simulink model "Model_CzasKroku"  (R2020b)
settings: Solver=VariableStepAuto  StartTime=0.0  StopTime=60  RelTol=1e-3
values from neighbouring files (symbols this model uses):
  g = 9.80665    [Strojenie_LQR_CzasKroku.m]    (also in Strojenie_LQR_Sila.m)
  K = lqr(A,B,Q,R)    [Strojenie_LQR_CzasKroku.m]    (also in Strojenie_LQR_Sila.m)
  L = 0.25    [Strojenie_LQR_CzasKroku.m]    (also in Strojenie_LQR_Sila.m)
  M = 1.5    [Strojenie_LQR_CzasKroku.m]    (also in Strojenie_LQR_Sila.m)
  m = 0.5    [Strojenie_LQR_CzasKroku.m]    (also in Strojenie_LQR_Sila.m)
settings Model: Creator=Maciej  LastModifiedBy=Maciej
settings DebuggingCC: AlgebraicLoopMsg=none

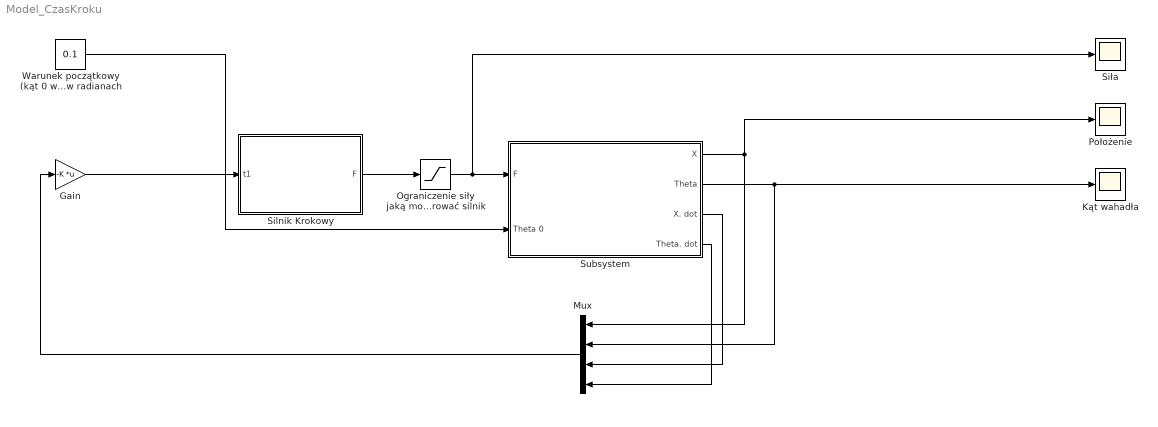
== system Model_CzasKroku ==
  Gain : Gain  Gain=-K  Multiplication=Matrix(K*u)
  Kąt wahadła : Scope
  Mux : Mux
  "Ograniczenie siły jaką może wygenerować silnik " : Saturate  UpperLimit=92  LowerLimit=-92
  Położenie : Scope
  Silnik Krokowy : Subsystem
  Siła : Scope
  Subsystem : Subsystem
  Warunek początkowy (kąt 0 wahadła) wyrażony w radianach : Constant  Value=0.1
  wires:
  Subsystem/1(X) -> Mux/1, Położenie/1
  Subsystem/2(Theta) -> Mux/2, Kąt wahadła/1
  Subsystem/3(X. dot) -> Mux/3
  Subsystem/4(Theta. dot) -> Mux/4
  Warunek początkowy (kąt 0 wahadła) wyrażony w radianach/1 -> Subsystem/2(Theta 0)
  "Ograniczenie siły jaką może wygenerować silnik "/1 -> Siła/1, Subsystem/1(F)
  Silnik Krokowy/1(F) -> "Ograniczenie siły jaką może wygenerować silnik "/1
  Mux/1 -> Gain/1
  Gain/1 -> Silnik Krokowy/1(t1)

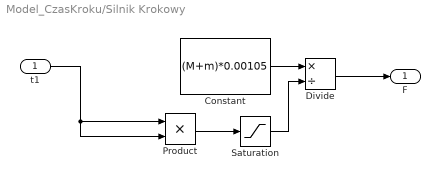
== system Model_CzasKroku/Silnik Krokowy ==
  t1 : Inport
  Constant : Constant  Value=(M+m)*0.00105
  Divide : Product  Inputs=*/
  Product : Product
  Saturation : Saturate  UpperLimit=inf  LowerLimit=0.001
  F : Outport
  wires:
  Constant/1 -> Divide/1
  Divide/1 -> F/1
  t1/1 -> Product/2, Product/1
  Product/1 -> Saturation/1
  Saturation/1 -> Divide/2

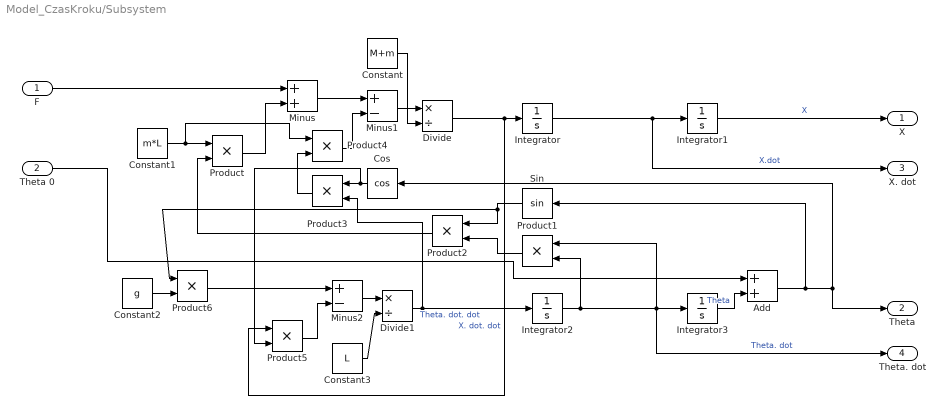
== system Model_CzasKroku/Subsystem ==
  F : Inport
  Theta 0 : Inport  Port=2
  Add : Sum
  Constant : Constant  Value=M+m
  Constant1 : Constant  Value=m*L
  Constant2 : Constant  Value=g
  Constant3 : Constant  Value=L
  Cos : Trigonometry  Operator=cos
  Divide : Product  Inputs=*/
  Divide1 : Product  Inputs=*/
  Integrator{,1..3} (4 alike) : Integrator
  Minus : Sum
  Minus1 : Sum  Inputs=+-
  Minus2 : Sum  Inputs=+-
  Product{,1..6} (7 alike) : Product
  Sin : Trigonometry
  X : Outport
  Theta : Outport  Port=2
  X. dot : Outport  Port=3
  Theta. dot : Outport  Port=4
  wires:
  Divide1/1 -> Product3/2, Integrator2/1  "Theta. dot. dot"
  Integrator3/1 -> Add/2  "Theta"
  Product5/1 -> Minus2/2
  Cos/1 -> Product5/2, Product3/1
  F/1 -> Minus/1
  Product2/1 -> Product/2
  Constant1/1 -> Product4/1, Product/1
  Constant3/1 -> Divide1/2
  Sin/1 -> Product6/1, Product2/1
  Constant/1 -> Divide/2
  Product4/1 -> Minus1/2
  Minus2/1 -> Divide1/1
  Divide/1 -> Product5/1, Integrator/1  "X. dot. dot"
  Product6/1 -> Minus2/1
  Integrator2/1 -> Product1/2, Theta. dot/1, Product1/1, Integrator3/1  "Theta. dot"
  Product/1 -> Minus/2
  Constant2/1 -> Product6/2
  Minus1/1 -> Divide/1
  Product1/1 -> Product2/2
  Product3/1 -> Product4/2
  Integrator/1 -> X. dot/1, Integrator1/1  "X.dot"
  Minus/1 -> Minus1/1
  Integrator1/1 -> X/1  "X"
  Add/1 -> Sin/1, Cos/1, Theta/1
  Theta 0/1 -> Add/1
